simulink model "sampleModel1991"  (R2023a)
settings: Solver=VariableStepAuto  StartTime=0.0  StopTime=10.0  RelTol=1e-3
libraries: hdlsllib x10
settings Model: Creator=user1  LastModifiedBy=user1

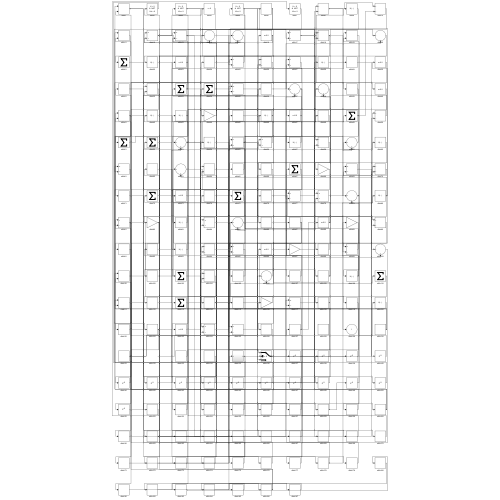
[thumbnail: Simulink's stored preview of the top-level diagram]
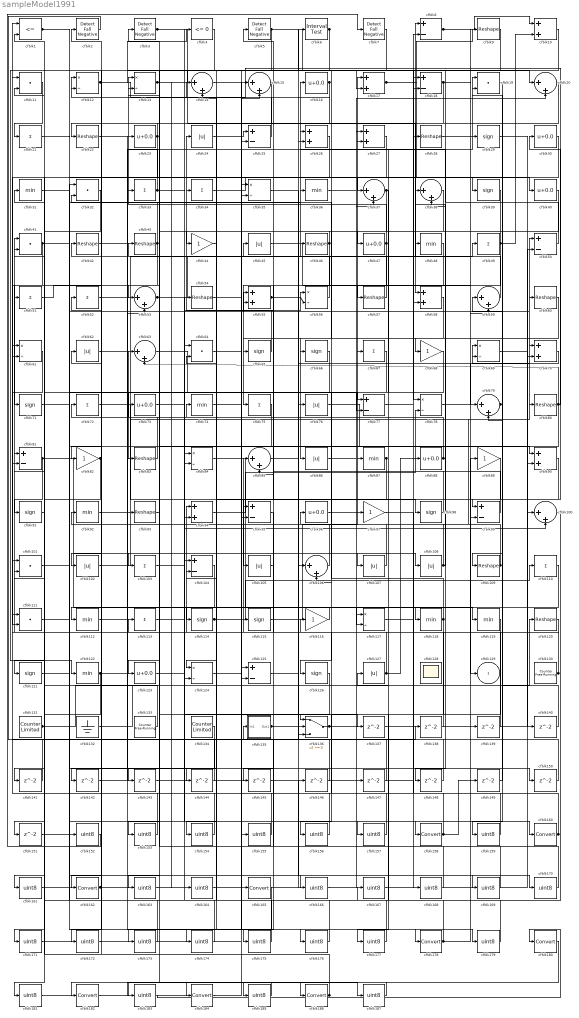
== system sampleModel1991 ==
  cfblk1 : RelationalOperator  Operator=<=  OutDataTypeStr=boolean  InputSameDT=off
  cfblk{10,17,26..27,55,58,70,90,94} (9 alike) : Sum
  cfblk{14..15,20,37..38,53,59,63,79,85,100,106} (12 alike) : Sum  Inputs=|++
  cfblk{11,19,32,41,64,101,111} (7 alike) : DotProduct  OutDataTypeStr=Inherit: Inherit via internal rule
  cfblk{24,45,62,76,86,102,105,107..108,127} (10 alike) : Abs  SaturateOnIntegerOverflow=off
  cfblk{21,33..34,49,51..52,67,72,75,103,110,113} (12 alike) : Sum  Inputs=+
  cfblk{8,18,25,50,77,81,95,99,104,125} (10 alike) : Sum  Inputs=+-
  cfblk{9,22,28,42..43,46,54,57,60,80,83,93,109,120} (14 alike) : Reshape
  cfblk{31,36,48,74,87,92,112,118..119,122} (10 alike) : MinMax
  cfblk{29,39,65..66,71,91,98,114..115,121,126} (11 alike) : Signum
  cfblk{44,68,82,89,97,116} (6 alike) : Gain
  cfblk{12..13,35,56,61,69,78,84,117,124} (10 alike) : Product  Inputs=*/  RndMeth=Zero  SaturateOnIntegerOverflow=on
  cfblk{16,23,30,40,47,73,88,96,123} (9 alike) : Bias  Bias=0.0  SaturateOnIntegerOverflow=off
  cfblk128 : Scope
      settings: Floating=on
  cfblk130 : hdlsllib/Sources/Counter Free-Running  NumBits=16  tsamp=-1
  cfblk131 : hdlsllib/Sources/Counter Limited  uplimit=7  tsamp=-1
  cfblk132 : Ground
  cfblk133 : hdlsllib/Sources/Counter Free-Running  NumBits=16  tsamp=-1
  cfblk134 : hdlsllib/Sources/Counter Limited  uplimit=7  tsamp=-1
  cfblk135 : Subsystem
      settings: LibrarySourceBlock=|
      | hdlsllib/Ports &
      | Subsystems/Subsystem
  cfblk136 : Switch  SaturateOnIntegerOverflow=off  InputSameDT=off
  cfblk{137..151} (15 alike) : Delay  SampleTime=1
  cfblk{152..157,159,161,163..164,166..177,179,181,183,185,187} (27 alike) : DataTypeConversion  OutDataTypeStr=uint8  SaturateOnIntegerOverflow=off  RndMeth=Floor
  cfblk{158,160,162,165,178,180,182,184,186} (9 alike) : DataTypeConversion  SaturateOnIntegerOverflow=off  RndMeth=Floor
  cfblk{2..3,5,7} (4 alike) : hdlsllib/Logic and Bit Operations/Detect Fall Negative  vinit=0  OutDataTypeStr=boolean
  cfblk4 : hdlsllib/Logic and Bit Operations/Compare To Zero  relop=<=  OutDataTypeStr=boolean
  cfblk6 : hdlsllib/Logic and Bit Operations/Interval Test  IntervalClosedRight=on  uplimit=0.5  IntervalClosedLeft=on  lowlimit=-0.5  OutDataTypeStr=boolean
  cfblk129 : Outport  VectorParamsAs1DForOutWhenUnconnected=off
  wires:
  cfblk107/1 -> cfblk17/1
  cfblk65/1 -> cfblk24/1
  cfblk120/1 -> cfblk41/1
  cfblk23/1 -> cfblk22/1, cfblk111/2
  cfblk130/1 -> cfblk94/1, cfblk5/1
  cfblk34/1 -> cfblk40/1
  cfblk58/1 -> cfblk86/1
  cfblk4/1 -> cfblk122/1
  cfblk110/1 -> cfblk112/1
  cfblk12/1 -> cfblk99/1, cfblk4/1, cfblk17/2
  cfblk73/1 -> cfblk56/1
  cfblk17/1 -> cfblk39/1, cfblk9/1
  cfblk84/1 -> cfblk118/1
  cfblk122/1 -> cfblk150/1, cfblk151/1
  cfblk59/1 -> cfblk16/1
  cfblk56/1 -> cfblk2/1
  cfblk28/1 -> cfblk19/1
  cfblk3/1 -> cfblk58/1, cfblk95/2
  cfblk46/1 -> cfblk44/1, cfblk95/1
  cfblk98/1 -> cfblk45/1
  cfblk13/1 -> cfblk20/1, cfblk164/1
  cfblk55/1 -> cfblk56/2, cfblk90/1
  cfblk85/1 -> cfblk76/1
  cfblk96/1 -> cfblk67/1
  cfblk37/1 -> cfblk77/1, cfblk174/1
  cfblk133/1 -> cfblk81/1
  cfblk8/1 -> cfblk79/1, cfblk10/1
  cfblk102/1 -> cfblk8/1
  cfblk109/1 -> cfblk50/1, cfblk14/2
  cfblk5/1 -> cfblk78/1, cfblk25/2, cfblk18/2
  cfblk47/1 -> cfblk13/1, cfblk57/1
  cfblk131/1 -> cfblk120/1, cfblk37/2
  cfblk117/1 -> cfblk119/1
  cfblk29/1 -> cfblk100/1
  cfblk92/1 -> cfblk80/1
  cfblk51/1 -> cfblk103/1
  cfblk21/1 -> cfblk37/1
  cfblk81/1 -> cfblk117/2, cfblk91/1
  cfblk45/1 -> cfblk99/2
  cfblk48/1 -> cfblk75/1
  cfblk112/1 -> cfblk29/1
  cfblk136/1 -> cfblk89/1, cfblk28/1
  cfblk43/1 -> cfblk71/1, cfblk32/2
  cfblk127/1 -> cfblk85/1, cfblk88/1
  cfblk94/1 -> cfblk78/2
  cfblk24/1 -> cfblk25/1
  cfblk105/1 -> cfblk55/1
  cfblk80/1 -> cfblk94/2, cfblk30/1, cfblk63/2
  cfblk108/1 -> cfblk96/1, cfblk38/1
  cfblk50/1 -> cfblk26/1
  cfblk75/1 -> cfblk123/1
  cfblk11/1 -> cfblk21/1
  cfblk52/1 -> cfblk178/1
  cfblk53/1 -> cfblk6/1, cfblk107/1
  cfblk115/1 -> cfblk87/1
  cfblk90/1 -> cfblk124/1
  cfblk77/1 -> cfblk49/1
  cfblk15/1 -> cfblk162/1
  cfblk76/1 -> cfblk129/1
  cfblk54/1 -> cfblk160/1
  cfblk57/1 -> cfblk46/1
  cfblk42/1 -> cfblk108/1
  cfblk121/1 -> cfblk55/2
  cfblk99/1 -> cfblk34/1
  cfblk72/1 -> cfblk98/1
  cfblk118/1 -> cfblk33/1, cfblk156/1
  cfblk68/1 -> cfblk83/1
  cfblk79/1 -> cfblk109/1, cfblk59/1
  cfblk63/1 -> cfblk125/1
  cfblk49/1 -> cfblk47/1, cfblk65/1, cfblk10/2
  cfblk82/1 -> cfblk121/1, cfblk142/1
  cfblk38/1 -> cfblk53/1
  cfblk114/1 -> cfblk110/1, cfblk115/1
  cfblk106/1 -> cfblk42/1
  cfblk20/1 -> cfblk102/1
  cfblk61/1 -> cfblk81/2
  cfblk39/1 -> cfblk68/1
  cfblk88/1 -> cfblk63/1, cfblk38/2
  cfblk135/1(Out1) -> cfblk106/1, cfblk175/1
  cfblk67/1 -> cfblk126/1
  cfblk86/1 -> cfblk48/1
  cfblk93/1 -> cfblk3/1
  cfblk25/1 -> cfblk12/1
  cfblk36/1 -> cfblk20/2
  cfblk62/1 -> cfblk93/1
  cfblk78/1 -> cfblk70/1
  cfblk7/1 -> cfblk66/1
  cfblk10/1 -> cfblk73/1
  cfblk89/1 -> cfblk105/1
  cfblk113/1 -> cfblk158/1
  cfblk26/1 -> cfblk51/1
  cfblk1/1 -> cfblk84/2, cfblk77/2
  cfblk44/1 -> cfblk14/1
  cfblk125/1 -> cfblk69/1
  cfblk83/1 -> cfblk72/1
  cfblk70/1 -> cfblk69/2
  cfblk132/1 -> cfblk26/2
  cfblk16/1 -> cfblk12/2, cfblk124/2
  cfblk123/1 -> cfblk100/2
  cfblk41/1 -> cfblk61/2, cfblk36/1
  cfblk33/1 -> cfblk23/1, cfblk90/2
  cfblk116/1 -> cfblk114/1
  cfblk87/1 -> cfblk106/2, cfblk136/3
  cfblk6/1 -> cfblk82/1, cfblk154/1
  cfblk18/1 -> cfblk125/2, cfblk59/2
  cfblk124/1 -> cfblk60/1
  cfblk14/1 -> cfblk136/1
  cfblk60/1 -> cfblk85/2
  cfblk103/1 -> cfblk137/1
  cfblk137/1 -> cfblk50/2
  cfblk2/1 -> cfblk138/1
  cfblk138/1 -> cfblk13/2
  cfblk139/1 -> cfblk11/1
  cfblk69/1 -> cfblk140/1
  cfblk140/1 -> cfblk79/2
  cfblk66/1 -> cfblk141/1
  cfblk141/1 -> cfblk1/1
  cfblk142/1 -> cfblk53/2
  cfblk31/1 -> cfblk143/1
  cfblk143/1 -> cfblk58/2
  cfblk30/1 -> cfblk144/1
  cfblk144/1 -> cfblk84/1
  cfblk95/1 -> cfblk145/1
  cfblk145/1 -> cfblk8/2
  cfblk146/1 -> cfblk136/2
  cfblk147/1 -> cfblk1/2
  cfblk9/1 -> cfblk148/1
  cfblk148/1 -> cfblk61/1
  cfblk149/1 -> cfblk19/2
  cfblk150/1 -> cfblk117/1
  cfblk101/1 -> cfblk152/1
  cfblk152/1 -> cfblk7/1
  cfblk126/1 -> cfblk153/1
  cfblk153/1 -> cfblk101/1
  cfblk154/1 -> cfblk101/2
  cfblk64/1 -> cfblk155/1
  cfblk155/1 -> cfblk41/2
  cfblk156/1 -> cfblk64/1
  cfblk151/1 -> cfblk157/1
  cfblk157/1 -> cfblk64/2
  cfblk158/1 -> cfblk149/1, cfblk111/1
  cfblk19/1 -> cfblk159/1
  cfblk159/1 -> cfblk113/1
  cfblk160/1 -> cfblk18/1, cfblk116/1
  cfblk32/1 -> cfblk161/1
  cfblk161/1 -> cfblk54/1
  cfblk162/1 -> cfblk147/1, cfblk146/1, cfblk70/2, cfblk62/1
  cfblk40/1 -> cfblk163/1
  cfblk163/1 -> cfblk15/1
  cfblk164/1 -> cfblk15/2
  cfblk22/1 -> cfblk166/1
  cfblk166/1 -> cfblk27/1
  cfblk100/1 -> cfblk167/1
  cfblk167/1 -> cfblk27/2
  cfblk97/1 -> cfblk168/1
  cfblk168/1 -> cfblk135/1(In1)
  cfblk71/1 -> cfblk169/1
  cfblk169/1 -> cfblk97/1
  cfblk35/1 -> cfblk170/1
  cfblk170/1 -> cfblk43/1
  cfblk91/1 -> cfblk171/1
  cfblk171/1 -> cfblk35/1
  cfblk134/1 -> cfblk172/1
  cfblk172/1 -> cfblk35/2
  cfblk104/1 -> cfblk173/1
  cfblk173/1 -> cfblk32/1
  cfblk174/1 -> cfblk104/1
  cfblk175/1 -> cfblk104/2
  cfblk74/1 -> cfblk176/1
  cfblk176/1 -> cfblk11/2
  cfblk119/1 -> cfblk177/1
  cfblk177/1 -> cfblk74/1
  cfblk178/1 -> cfblk139/1, cfblk127/1
  cfblk111/1 -> cfblk179/1
  cfblk179/1 -> cfblk52/1
  cfblk27/1 -> cfblk181/1
  cfblk181/1 -> cfblk165/1
  cfblk165/1 -> cfblk183/1
  cfblk183/1 -> cfblk180/1
  cfblk184/1 -> cfblk186/1
  cfblk180/1 -> cfblk185/1
  cfblk185/1 -> cfblk182/1
  cfblk186/1 -> cfblk92/1, cfblk31/1
  cfblk182/1 -> cfblk187/1
  cfblk187/1 -> cfblk184/1

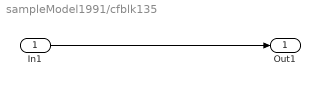
== system sampleModel1991/cfblk135 ==
  In1 : Inport
  Out1 : Outport
  wires:
  In1/1 -> Out1/1
